simulink model "proyecto_Parkinson_LazoCerrado"  (R2024b)
settings: Solver=VariableStepAuto  StartTime=0.0  StopTime=10.0  RelTol=1e-3
libraries: slpidlib x1
settings Model: Creator=Dario  LastModifiedBy=Dario

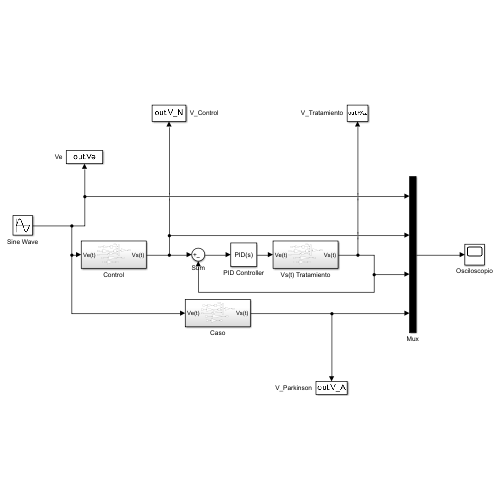
[thumbnail: Simulink's stored preview of the top-level diagram]
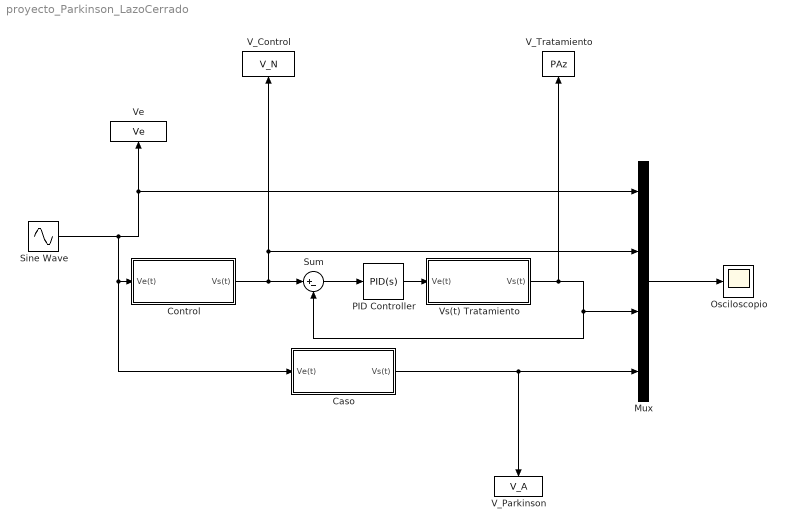
== system proyecto_Parkinson_LazoCerrado ==
  Caso : Subsystem
  Control : Subsystem
  Mux : Mux
  Osciloscopio : Scope
  PID Controller : slpidlib/PID Controller  Controller=PID  Form=Parallel  TimeDomain=Continuous-time  UseExternalTs=off  SampleTime=-1  IntegratorMethod=Forward Euler  FilterMethod=Forward Euler  ControllerParametersSource=internal  P=0  I=67265.6401452196  UseKiTs=off  D=0  UseExternalDerivativeSource=off  N=100  UseFilter=on  TunerSelectOption=Transfer Function Based (PID Tuner App)  InitialConditionSource=internal  InitialConditionForIntegrator=0  InitialConditionForFilter=0  DifferentiatorICPrevScaledInput=0  ExternalReset=none  TrackingMode=off  Kt=1  LimitOutput=off  SatLimitsSource=internal  UpperSaturationLimit=inf  LowerSaturationLimit=-inf  LinearizeAsGain=on  AntiWindupMode=none  Kb=1  LimitIntegrator=off  UpperIntegratorSaturationLimit=inf  LowerIntegratorSaturationLimit=-inf  POutMin=[]  POutMax=[]  IOutMin=[]  IOutMax=[]  DOutMin=[]  DOutMax=[]  NOutMin=[]  NOutMax=[]  SumOutMin=[]  SumOutMax=[]  SaturationOutMin=[]  SaturationOutMax=[]  PParamMin=[]  PParamMax=[]  IParamMin=[]  IParamMax=[]  DParamMin=[]  DParamMax=[]  NParamMin=[]  NParamMax=[]  KbParamMin=[]  KbParamMax=[]  KtParamMin=[]  KtParamMax=[]  KbOutMin=[]  KbOutMax=[]  KtOutMin=[]  KtOutMax=[]  IntegratorOutMin=[]  IntegratorOutMax=[]  FilterOutMin=[]  FilterOutMax=[]  SumI1OutMin=[]  SumI1OutMax=[]  SumI2OutMin=[]  SumI2OutMax=[]  SumI3OutMin=[]  SumI3OutMax=[]  SumI4OutMin=[]  SumI4OutMax=[]  SumDOutMin=[]  SumDOutMax=[]  DifferentiatorOutMin=[]  DifferentiatorOutMax=[]  FilterDiffOutCoefMin=[]  FilterDiffOutCoefMax=[]  ReciprocalOutMin=[]  ReciprocalOutMax=[]  SumDenOutMin=[]  SumDenOutMax=[]  SumNumOutMin=[]  SumNumOutMax=[]  DivideOutMin=[]  DivideOutMax=[]  UdiffTsProdOutMin=[]  UdiffTsProdOutMax=[]  NTsProdOutMin=[]  NTsProdOutMax=[]  UintegralTsProdOutMin=[]  UintegralTsProdOutMax=[]  UngainTsProdOutMin=[]  UngainTsProdOutMax=[]  ClampingZeroOutDataTypeStr=Inherit: Inherit via back propagation  ClampingZeroOutMin=[]  ClampingZeroOutMax=[]  FilterDenConstantOutDataTypeStr=Inherit: Inherit via back propagation  FilterDenConstantOutMin=[]  FilterDenConstantOutMax=[]  PCopyOutDataTypeStr=Inherit: Inherit via back propagation  PCopyOutMin=[]  PCopyOutMax=[]  NCopyOutDataTypeStr=Inherit: Inherit via back propagation  NCopyOutMin=[]  NCopyOutMax=[]  IntegratorContinuousStateAttributes=''  IntegratorStateMustResolveToSignalObject=off  IntegratorRTWStateStorageClass=Auto  FilterContinuousStateAttributes=''  FilterStateMustResolveToSignalObject=off  FilterRTWStateStorageClass=Auto  ParallelPVariant=InternalParameters  IdealPVariant=Disabled  IVariant=InternalParameters  DVariant=InternalParameters  IntegratorVariant=Continuous  SatVariant=Disabled  AWVariant=Passthrough  PCopyVariant=Disabled  TRVariant=Disabled  FdbkBlocksVariant=Forward  IdealPFdbkVariant=Disabled  SatFdbkVariant=Disabled  DerivativeFilterVariant=ContFilter  NVariant=InternalParameters  NCopyVariant=Disabled  FilterICVariant=InternalICsFilter  IntegratorICVariant=InternalICs  ExternalResetVariant=Disabled  TRSumVariant=Passthrough  SumFdbkVariant=Disabled  SumVariant=Sum_PID  TsampFilterVariant=InternalTs  TsampNgainVariant=Passthrough  TsampIntegralVariant=Disabled_SignalSpec  ExternalSaturationOutDataTypeStr=Inherit: Same as second input  DerivativeSourceVariant=ErrorSignal  PreIntVariant=InternalPreInt
  Sine Wave : Sin  Amplitude=5  Frequency=4  SampleTime=0
  Sum : Sum  Inputs=|+-
  V_Control : ToWorkspace  VariableName=V_N  SampleTime=-1
  V_Parkinson : ToWorkspace  VariableName=V_A  SampleTime=-1
  V_Tratamiento : ToWorkspace  VariableName=PAz  SampleTime=-1
  Ve : ToWorkspace  VariableName=Ve  SampleTime=-1
      settings: Tag=Ve
  Vs(t) Tratamiento : Subsystem
  wires:
  Sine Wave/1 -> Mux/1, Ve/1, Caso/1(Ve(t)), Control/1(Ve(t))
  Mux/1 -> Osciloscopio/1
  Control/1(Vs(t)) -> Mux/2, V_Control/1, Sum/1
  Caso/1(Vs(t)) -> V_Parkinson/1, Mux/4
  Sum/1 -> PID Controller/1
  PID Controller/1 -> Vs(t) Tratamiento/1(Ve(t))
  Vs(t) Tratamiento/1(Vs(t)) -> Sum/2, Mux/3, V_Tratamiento/1

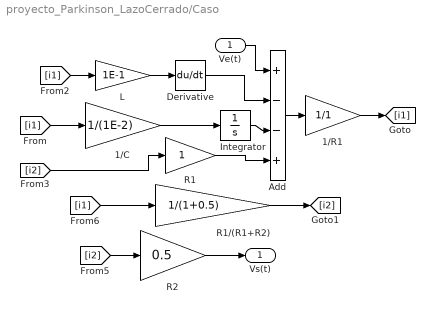
== system proyecto_Parkinson_LazoCerrado/Caso ==
  Ve(t) : Inport
  1/C : Gain  Gain=1/(1E-2)
  1/R1 : Gain  Gain=1/1
  Add : Sum  Inputs=+--+
  Derivative : Derivative
  Integrator : Integrator
  L : Gain  Gain=1E-1
  R1 : Gain
  R1/(R1+R2) : Gain  Gain=1/(1+0.5)
  R2 : Gain  Gain=0.5
  Vs(t) : Outport
  wires:
  [i1] -> L/1
  Derivative/1 -> Add/2
  Add/1 -> 1/R1/1
  1/C/1 -> Integrator/1
  R1/(R1+R2)/1 -> [i2]
  [i2] -> R2/1
  R2/1 -> Vs(t)/1
  1/R1/1 -> [i1]
  Ve(t)/1 -> Add/1
  Integrator/1 -> Add/3
  R1/1 -> Add/4
  [i2] -> R1/1
  [i1] -> 1/C/1
  L/1 -> Derivative/1
  [i1] -> R1/(R1+R2)/1

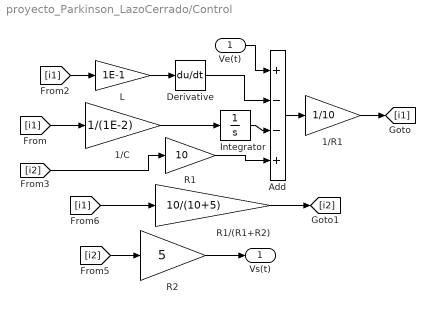
== system proyecto_Parkinson_LazoCerrado/Control ==
  Ve(t) : Inport
  1/C : Gain  Gain=1/(1E-2)
  1/R1 : Gain  Gain=1/10
  Add : Sum  Inputs=+--+
  Derivative : Derivative
  Integrator : Integrator
  L : Gain  Gain=1E-1
  R1 : Gain  Gain=10
  R1/(R1+R2) : Gain  Gain=10/(10+5)
  R2 : Gain  Gain=5
  Vs(t) : Outport
  wires:
  Integrator/1 -> Add/3
  [i2] -> R2/1
  R2/1 -> Vs(t)/1
  1/R1/1 -> [i1]
  Ve(t)/1 -> Add/1
  [i1] -> 1/C/1
  [i2] -> R1/1
  [i1] -> R1/(R1+R2)/1
  R1/1 -> Add/4
  L/1 -> Derivative/1
  1/C/1 -> Integrator/1
  Derivative/1 -> Add/2
  [i1] -> L/1
  Add/1 -> 1/R1/1
  R1/(R1+R2)/1 -> [i2]

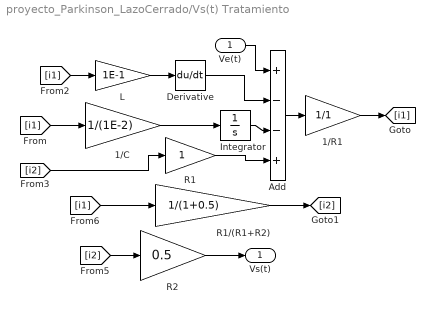
== system proyecto_Parkinson_LazoCerrado/Vs(t) Tratamiento ==
  Ve(t) : Inport
  1/C : Gain  Gain=1/(1E-2)
  1/R1 : Gain  Gain=1/1
  Add : Sum  Inputs=+--+
  Derivative : Derivative
  Integrator : Integrator
  L : Gain  Gain=1E-1
  R1 : Gain
  R1/(R1+R2) : Gain  Gain=1/(1+0.5)
  R2 : Gain  Gain=0.5
  Vs(t) : Outport
  wires:
  [i1] -> L/1
  Derivative/1 -> Add/2
  Add/1 -> 1/R1/1
  1/C/1 -> Integrator/1
  R1/(R1+R2)/1 -> [i2]
  [i2] -> R2/1
  R2/1 -> Vs(t)/1
  1/R1/1 -> [i1]
  Ve(t)/1 -> Add/1
  Integrator/1 -> Add/3
  R1/1 -> Add/4
  [i2] -> R1/1
  [i1] -> 1/C/1
  L/1 -> Derivative/1
  [i1] -> R1/(R1+R2)/1
